simulink model "Aerodynamic_11"  (R2022b)
settings: Solver=FixedStepDiscrete  StartTime=0.0  StopTime=1  FixedStep=1  RelTol=1e-3
values from neighbouring files (symbols this model uses):
  e_input = input('Enter the value of e ')    [Test1.m]
  v_input = input('Enter value of V ')    [Test1.m]
settings Model: Creator=horty  LastModifiedBy=horty

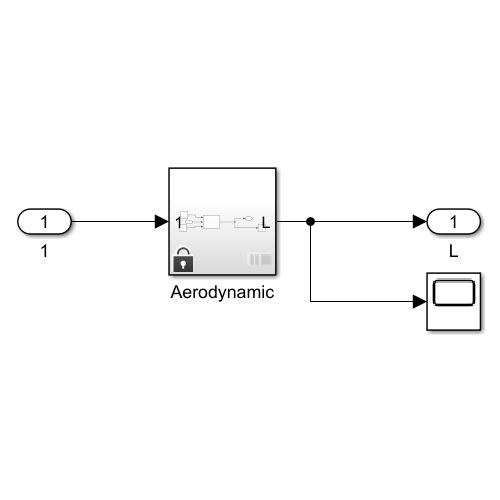
[thumbnail: Simulink's stored preview of the top-level diagram]
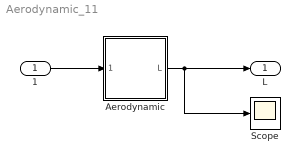
== system Aerodynamic_11 ==
  1 : Inport
  Aerodynamic : Subsystem
  Scope : Scope
  L : Outport
  wires:
  1/1 -> Aerodynamic/1(1)
  Aerodynamic/1(L) -> L/1, Scope/1

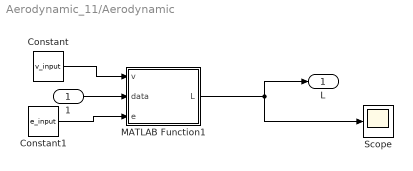
== system Aerodynamic_11/Aerodynamic ==
  1 : Inport
  Constant : Constant  Value=v_input
  Constant1 : Constant  Value=e_input
  MATLAB Function1 : MATLAB Function  TreatAsAtomicUnit=on
  Scope : Scope
  L : Outport
  wires:
  MATLAB Function1/1(L) -> L/1, Scope/1
  Constant/1 -> MATLAB Function1/1(v)
  Constant1/1 -> MATLAB Function1/3(e)
  1/1 -> MATLAB Function1/2(data)

== matlab function Aerodynamic_11/Aerodynamic/MATLAB Function1 ==
  data: v input; data input; e input; L output
function L = fcn(v,data,e)
data=1;
Cl=0.01;
S=100;
L=1/2*e*Cl*S*(v^2);
